simulink model "EV_powertrain"  (R2018a)
settings: Solver=FixedStepAuto  StartTime=0.0  StopTime=10.5  FixedStep=0.1  MaxStep=19.86  RelTol=1e-3
values from neighbouring files (symbols this model uses):
  A = 3.8065    [artemisUrban_drive_cycle.m]
  cd = 0.28    [artemisUrban_drive_cycle.m]
  crf = 0.015    [artemisUrban_drive_cycle.m]
  GR = 7.9377    [artemisUrban_drive_cycle.m]
  GVM = M+Md    (= 1710.665)    [artemisUrban_drive_cycle.m]
  GVW = GVM*g    (= 16781.62365)    [artemisUrban_drive_cycle.m]
  MCE_Eff = MCE(:,2:16)    [artemisUrban_drive_cycle.m]
  MCE_Speed = MCE(:,1)    [artemisUrban_drive_cycle.m]
  MCE_Torque = MCE(:,17)    [artemisUrban_drive_cycle.m]
  MCRE_Eff = MCRE(:,2:16)    [artemisUrban_drive_cycle.m]
  MCRE_Speed = MCRE(:,1)    [artemisUrban_drive_cycle.m]
  MCRE_Torque = MCRE(:,17)    [artemisUrban_drive_cycle.m]
  ME_Eff = ME(:,2:16)    [artemisUrban_drive_cycle.m]
  ME_Speed = ME(:,1)    [artemisUrban_drive_cycle.m]
  ME_Torque = ME(:,17)    [artemisUrban_drive_cycle.m]
  MRE_Eff = MRE(:,2:16)    [artemisUrban_drive_cycle.m]
  MRE_Speed = MRE(:,1)    [artemisUrban_drive_cycle.m]
  MRE_Torque = MRE(:,17)    [artemisUrban_drive_cycle.m]
  rho = 1.2250    (= 1.225)    [artemisUrban_drive_cycle.m]
  Rw = 0.2032    [artemisUrban_drive_cycle.m]
  Teff = 0.89    [artemisUrban_drive_cycle.m]
settings Model: Creator=VAISHNAV  LastModifiedBy=VAISHNAV

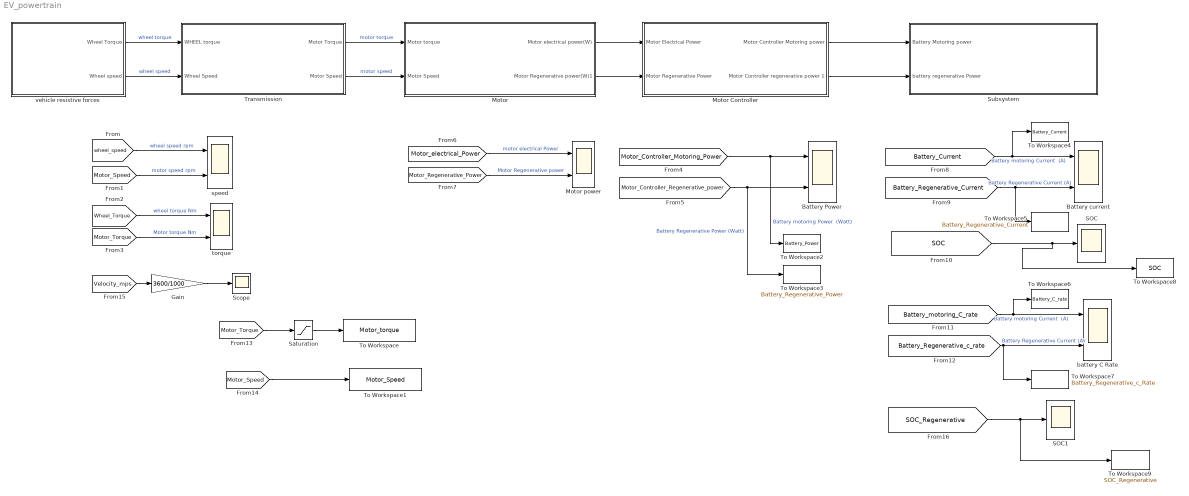
== system EV_powertrain ==
  Battery Power : Scope  NumInputPorts=2
  "Battery current " : Scope  NumInputPorts=2
  Gain : Gain  Gain=3600/1000
  "Motor " : Subsystem
  Motor Controller : Subsystem
  Motor power : Scope  NumInputPorts=2
  SOC : Scope
  SOC1 : Scope
  Saturation : Saturate  UpperLimit=inf  LowerLimit=0
  Scope : Scope
  Subsystem : Subsystem
  To Workspace : ToWorkspace  VariableName=Motor_torque  SaveFormat=Timeseries  SampleTime=-1
  To Workspace1 : ToWorkspace  VariableName=Motor_Speed  SaveFormat=Timeseries  SampleTime=-1
  To Workspace2 : ToWorkspace  VariableName=Battery_Power  SaveFormat=Timeseries  SampleTime=-1
  To Workspace3 : ToWorkspace  VariableName=Battery_Regenerative_Power  SaveFormat=Timeseries  SampleTime=-1
  To Workspace4 : ToWorkspace  VariableName=Battery_Current  SaveFormat=Timeseries  SampleTime=-1
  To Workspace5 : ToWorkspace  VariableName=Battery_Regenerative_Current  SaveFormat=Timeseries  SampleTime=-1
  To Workspace6 : ToWorkspace  VariableName=Battery_C_rate  SaveFormat=Timeseries  SampleTime=-1
  To Workspace7 : ToWorkspace  VariableName=Battery_Regenerative_c_Rate  SaveFormat=Timeseries  SampleTime=-1
  To Workspace8 : ToWorkspace  VariableName=SOC  SaveFormat=Timeseries  SampleTime=-1
  To Workspace9 : ToWorkspace  VariableName=SOC_Regenerative  SaveFormat=Timeseries  SampleTime=-1
  Transmission : Subsystem
  battery C Rate : Scope  NumInputPorts=2
  speed : Scope  NumInputPorts=2
  torque : Scope  NumInputPorts=2
  vehicle resistive forces : Subsystem
  wires:
  vehicle resistive forces/1(Wheel Torque) -> Transmission/1(WHEEL torque)  "wheel torque"
  vehicle resistive forces/2(Wheel speed) -> Transmission/2(Wheel Speed)  "wheel speed"
  [wheel_speed] -> speed/1  "wheel speed rpm"
  [Motor_Speed] -> speed/2  "motor speed rpm"
  [Wheel_Torque] -> torque/1  "wheel torque Nm"
  [Motor_Torque] -> torque/2  "Motor torque Nm"
  Transmission/1(Motor Torque) -> "Motor "/1(Motor torque)  "motor torque"
  Transmission/2(Motor Speed) -> "Motor "/2(Motor Speed)  "motor speed"
  [Motor_electrical_Power] -> Motor power/1  "motor electrical Power"
  [Motor_Regenerative_Power] -> Motor power/2  "Motor Regenerative power"
  "Motor "/1(Motor electrical power(W)) -> Motor Controller/1(Motor Electrical Power)
  "Motor "/2(Motor Regenerative power(W)1) -> Motor Controller/2(Motor Regenerative Power)
  [Motor_Controller_Motoring_Power] -> To Workspace2/1, Battery Power/1  "Battery motoring Power  (Watt)"
  [Motor_Controller_Regenerative_power] -> To Workspace3/1, Battery Power/2  "Battery Regenerative Power (Watt)"
  [Battery_Current] -> To Workspace4/1, "Battery current "/1  "Battery motoring Current  (A)"
  [Battery_Regenerative_Current] -> To Workspace5/1, "Battery current "/2  "Battery Regenerative Current (A)"
  [SOC] -> To Workspace8/1, SOC/1
  [Battery_Regenerative_c_rate] -> To Workspace7/1, battery C Rate/2  "Battery Regenerative Current (A)"
  [Battery_motoring_C_rate] -> To Workspace6/1, battery C Rate/1  "Battery motoring Current  (A)"
  Saturation/1 -> To Workspace/1
  [Motor_Torque] -> Saturation/1
  [Motor_Speed] -> To Workspace1/1
  [Velocity_mps] -> Gain/1
  Gain/1 -> Scope/1
  [SOC_Regenerative] -> To Workspace9/1, SOC1/1
  Motor Controller/2(Motor Controller regenerative power 1) -> Subsystem/2(battery regenerative Power)
  Motor Controller/1("Motor Controller Motoring power ") -> Subsystem/1(Battery Motoring power)

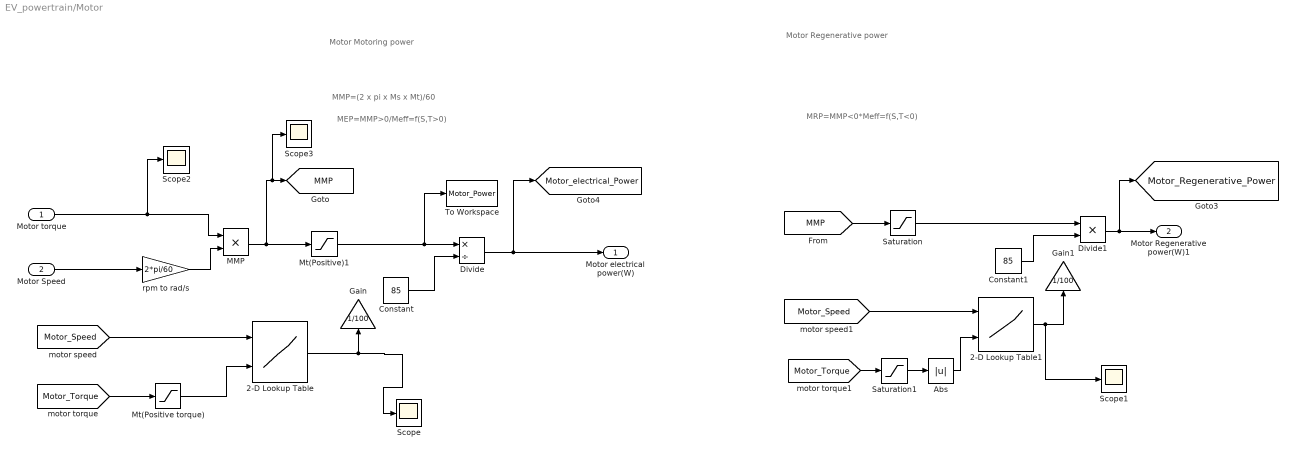
== system EV_powertrain/Motor  ==
  note: MRP=MMP<0*Meff=f(S,T<0)
  note: Motor Regenerative power
  note: MEP=MMP>0/Meff=f(S,T>0)
  note: MMP=(2 x pi x Ms x Mt)/60
  note: Motor Motoring power
  Motor torque : Inport
  Motor Speed : Inport  Port=2
  2-D Lookup Table : Lookup_n-D  BreakpointsForDimension1=ME_Speed  BreakpointsForDimension2=ME_Torque  Table=ME_Eff  InternalRulePriority=Speed  RndMeth=Simplest  InputSameDT=on
  2-D Lookup Table1 : Lookup_n-D  BreakpointsForDimension1=MRE_Speed  BreakpointsForDimension2=MRE_Torque  Table=MRE_Eff  InternalRulePriority=Speed  RndMeth=Simplest  InputSameDT=on
  Abs : Abs
  Constant : Constant  Value=85
  Constant1 : Constant  Value=85
  Divide : Product  Inputs=*/
  Divide1 : Product  Inputs=**
  Gain : Gain  Gain=1/100
  Gain1 : Gain  Gain=1/100
  MMP : Product
  Mt(Positive torque) : Saturate  UpperLimit=inf  LowerLimit=0
  Mt(Positive)1 : Saturate  UpperLimit=inf  LowerLimit=0
  Saturation : Saturate  UpperLimit=0  LowerLimit=-inf
  Saturation1 : Saturate  UpperLimit=0  LowerLimit=-inf
  Scope{,1..3} (4 alike) : Scope
  To Workspace : ToWorkspace  VariableName=Motor_Power  SaveFormat=Timeseries  SampleTime=-1
  rpm to rad/s : Gain  Gain=2*pi/60
  Motor electrical power(W) : Outport
  Motor Regenerative power(W)1 : Outport  Port=2
  tag scope: MMP=global, Motor_Regenerative_Power=global, Motor_electrical_Power=global
  wires:
  Motor Speed/1 -> rpm to rad/s/1
  Motor torque/1 -> Scope2/1, MMP/1
  rpm to rad/s/1 -> MMP/2
  [Motor_Speed] -> 2-D Lookup Table/1
  Mt(Positive torque)/1 -> 2-D Lookup Table/2
  [Motor_Torque] -> Mt(Positive torque)/1
  MMP/1 -> Scope3/1, [MMP], Mt(Positive)1/1
  Divide/1 -> [Motor_electrical_Power], Motor electrical power(W)/1
  Mt(Positive)1/1 -> To Workspace/1, Divide/1
  [MMP] -> Saturation/1
  [Motor_Torque] -> Saturation1/1
  [Motor_Speed] -> 2-D Lookup Table1/1
  2-D Lookup Table1/1 -> Scope1/1, Gain1/1
  Saturation/1 -> Divide1/1
  Saturation1/1 -> Abs/1
  Abs/1 -> 2-D Lookup Table1/2
  Divide1/1 -> [Motor_Regenerative_Power], Motor Regenerative power(W)1/1
  2-D Lookup Table/1 -> Scope/1, Gain/1
  Constant/1 -> Divide/2
  Constant1/1 -> Divide1/2

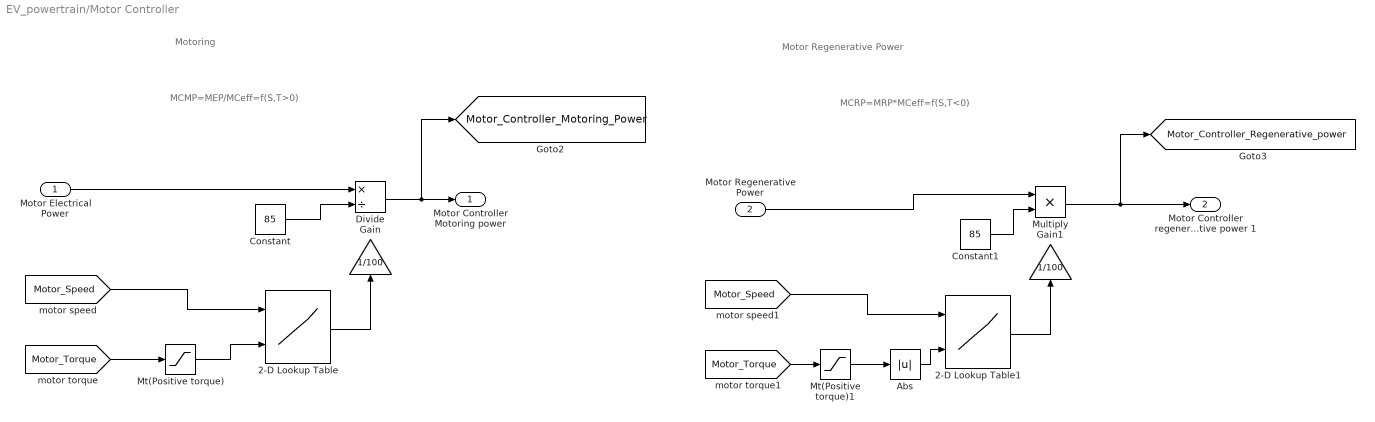
== system EV_powertrain/Motor Controller ==
  note: MCRP=MRP*MCeff=f(S,T<0)
  note: Motor Regenerative Power
  note: MCMP=MEP/MCeff=f(S,T>0)
  note: Motoring
  Motor Electrical Power : Inport
  Motor Regenerative Power : Inport  Port=2
  2-D Lookup Table : Lookup_n-D  BreakpointsForDimension1=MCE_Speed  BreakpointsForDimension2=MCE_Torque  Table=MCE_Eff  InternalRulePriority=Speed  RndMeth=Simplest  InputSameDT=on
  2-D Lookup Table1 : Lookup_n-D  BreakpointsForDimension1=MCRE_Speed  BreakpointsForDimension2=MCRE_Torque  Table=MCRE_Eff  InternalRulePriority=Speed  RndMeth=Simplest  InputSameDT=on
  Abs : Abs
  Constant : Constant  Value=85
  Constant1 : Constant  Value=85
  Divide : Product  Inputs=*/
  Gain : Gain  Gain=1/100
  Gain1 : Gain  Gain=1/100
  Mt(Positive torque) : Saturate  UpperLimit=inf  LowerLimit=0
  Mt(Positive torque)1 : Saturate  UpperLimit=0  LowerLimit=-inf
  Multiply : Product
  "Motor Controller Motoring power " : Outport
  Motor Controller regenerative power 1 : Outport  Port=2
  tag scope: Motor_Controller_Motoring_Power=global, Motor_Controller_Regenerative_power=global
  wires:
  [Motor_Torque] -> Mt(Positive torque)/1
  [Motor_Speed] -> 2-D Lookup Table/1
  Mt(Positive torque)/1 -> 2-D Lookup Table/2
  2-D Lookup Table/1 -> Gain/1
  Motor Electrical Power/1 -> Divide/1
  Divide/1 -> [Motor_Controller_Motoring_Power], "Motor Controller Motoring power "/1
  [Motor_Speed] -> 2-D Lookup Table1/1
  [Motor_Torque] -> Mt(Positive torque)1/1
  2-D Lookup Table1/1 -> Gain1/1
  Motor Regenerative Power/1 -> Multiply/1
  Multiply/1 -> [Motor_Controller_Regenerative_power], Motor Controller regenerative power 1/1
  Mt(Positive torque)1/1 -> Abs/1
  Abs/1 -> 2-D Lookup Table1/2
  Constant/1 -> Divide/2
  Constant1/1 -> Multiply/2

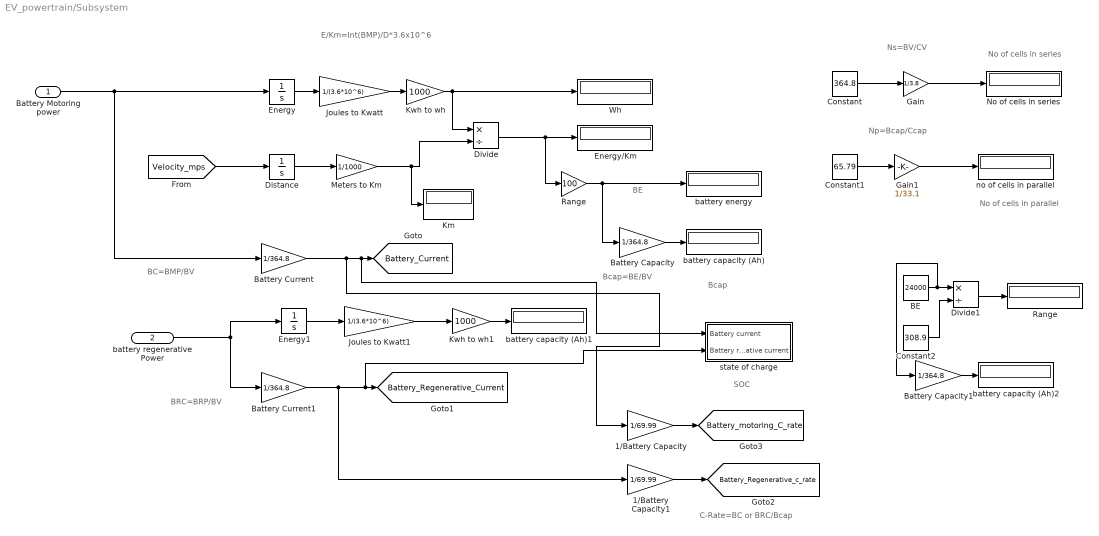
== system EV_powertrain/Subsystem ==
  note: BC=BMP/BV
  note: Bcap
  note: BE
  note: No of cells in parallel
  note: No of cells in series
  note: C-Rate=BC or BRC/Bcap
  note: SOC
  note: Np=Bcap/Ccap
  note: Ns=BV/CV
  note: Bcap=BE/BV
  note: E/Km=Int(BMP)/D*3.6x10^6
  note: BRC=BRP/BV
  Battery Motoring power : Inport
  battery regenerative Power : Inport  Port=2
  1/Battery Capacity : Gain  Gain=1/69.99
  1/Battery Capacity1 : Gain  Gain=1/69.99
  BE : Constant  Value=24000
  Battery Capacity : Gain  Gain=1/364.8
  Battery Capacity1 : Gain  Gain=1/364.8
  Battery Current : Gain  Gain=1/364.8
  Battery Current1 : Gain  Gain=1/364.8
  Constant : Constant  Value=364.8
  Constant1 : Constant  Value=65.79
  Constant2 : Constant  Value=308.9
  Distance : Integrator
  Divide : Product  Inputs=*/
  Divide1 : Product  Inputs=*/
  Energy : Integrator
  Energy/Km : Display
  Energy1 : Integrator
  Gain : Gain  Gain=1/3.8
  Gain1 : Gain  Gain=1/33.1
  Joules to Kwatt : Gain  Gain=1/(3.6*10^6)
  Joules to Kwatt1 : Gain  Gain=1/(3.6*10^6)
  Km : Display
  Kwh to wh : Gain  Gain=1000
  Kwh to wh1 : Gain  Gain=1000
  Meters to Km : Gain  Gain=1/1000
  No of cells in series : Display
  Range : Gain  Gain=100
  "Range " : Display
  Wh : Display
  battery capacity (Ah) : Display
  battery capacity (Ah)1 : Display
  battery capacity (Ah)2 : Display
  battery energy : Display
  no of cells in parallel : Display
  state of charge : Subsystem
  tag scope: Battery_Current=global, Battery_Regenerative_Current=global, Battery_Regenerative_c_rate=global, Battery_motoring_C_rate=global
  wires:
  Battery Motoring power/1 -> Energy/1, Battery Current/1
  [Velocity_mps] -> Distance/1
  Energy/1 -> Joules to Kwatt/1
  Joules to Kwatt/1 -> Kwh to wh/1
  Kwh to wh/1 -> Wh/1, Divide/1
  Divide/1 -> Range/1, Energy/Km/1
  Distance/1 -> Meters to Km/1
  Meters to Km/1 -> Km/1, Divide/2
  Range/1 -> Battery Capacity/1, battery energy/1
  Battery Capacity/1 -> battery capacity (Ah)/1
  battery regenerative Power/1 -> Energy1/1, Battery Current1/1
  Battery Current1/1 -> 1/Battery Capacity1/1, state of charge/2("Battery regenerative current "), [Battery_Regenerative_Current]
  Energy1/1 -> Joules to Kwatt1/1
  Joules to Kwatt1/1 -> Kwh to wh1/1
  Kwh to wh1/1 -> battery capacity (Ah)1/1
  Gain/1 -> No of cells in series/1
  Constant/1 -> Gain/1
  Constant1/1 -> Gain1/1
  Gain1/1 -> no of cells in parallel/1
  1/Battery Capacity/1 -> [Battery_motoring_C_rate]
  1/Battery Capacity1/1 -> [Battery_Regenerative_c_rate]
  Constant2/1 -> Divide1/2
  BE/1 -> Battery Capacity1/1, Divide1/1
  Divide1/1 -> "Range "/1
  Battery Capacity1/1 -> battery capacity (Ah)2/1
  Battery Current/1 -> 1/Battery Capacity/1, state of charge/1(Battery current), [Battery_Current]

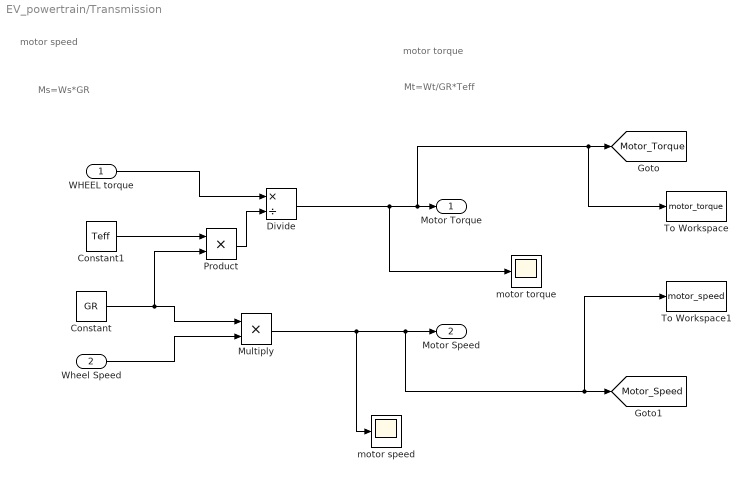
== system EV_powertrain/Transmission ==
  note: Mt=Wt/GR*Teff
  note: Ms=Ws*GR
  note: motor torque
  note: motor speed
  WHEEL torque : Inport
  Wheel Speed : Inport  Port=2
  Constant : Constant  Value=GR
  Constant1 : Constant  Value=Teff
  Divide : Product  Inputs=*/
  Multiply : Product
  Product : Product
  To Workspace : ToWorkspace  VariableName=motor_torque  SaveFormat=Timeseries  SampleTime=-1
  To Workspace1 : ToWorkspace  VariableName=motor_speed  SaveFormat=Timeseries  SampleTime=-1
  motor speed : Scope
  motor torque : Scope
  Motor Torque : Outport
  Motor Speed : Outport  Port=2
  tag scope: Motor_Speed=global, Motor_Torque=global
  wires:
  Wheel Speed/1 -> Multiply/2
  Constant/1 -> Product/2, Multiply/1
  Multiply/1 -> motor speed/1, To Workspace1/1, [Motor_Speed], Motor Speed/1
  Divide/1 -> motor torque/1, To Workspace/1, [Motor_Torque], Motor Torque/1
  Constant1/1 -> Product/1
  Product/1 -> Divide/2
  WHEEL torque/1 -> Divide/1

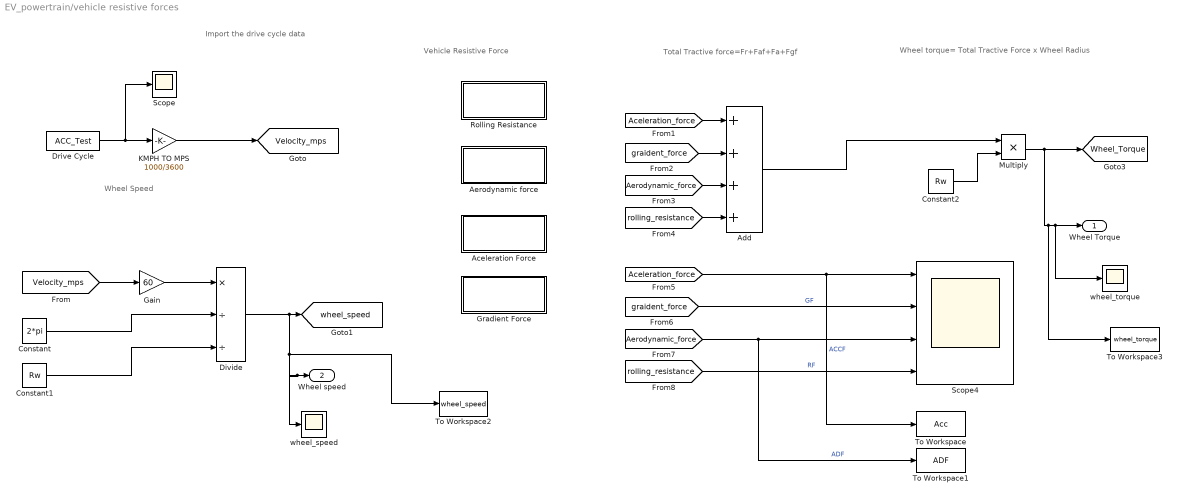
== system EV_powertrain/vehicle resistive forces ==
  note: Wheel torque= Total Tractive Force x Wheel Radius
  note: Total Tractive force=Fr+Faf+Fa+Fgf
  note: Vehicle Resistive Force
  note: Wheel Speed
  note: Import the drive cycle data
  Aceleration Force : Subsystem
  Add : Sum  Inputs=++++
  Aerodynamic force : Subsystem
  Constant : Constant  Value=2*pi
  Constant1 : Constant  Value=Rw
  Constant2 : Constant  Value=Rw
  Divide : Product  Inputs=*//
  Drive Cycle : FromWorkspace  VariableName=ACC_Test  SampleTime=0
  Gain : Gain  Gain=60
  Gradient Force : Subsystem
  KMPH TO MPS : Gain  Gain=1000/3600
  Multiply : Product
  Rolling Resistance : Subsystem
  Scope : Scope
  Scope4 : Scope  NumInputPorts=4
  To Workspace : ToWorkspace  VariableName=Acc  SaveFormat=Timeseries  SampleTime=-1
  To Workspace1 : ToWorkspace  VariableName=ADF  SaveFormat=Timeseries  SampleTime=-1
  To Workspace2 : ToWorkspace  VariableName=wheel_speed  SaveFormat=Timeseries  SampleTime=-1
  To Workspace3 : ToWorkspace  VariableName=wheel_torque  SaveFormat=Timeseries  SampleTime=-1
  wheel_speed : Scope
  wheel_torque : Scope
  Wheel Torque : Outport
  Wheel speed : Outport  Port=2
  tag scope: Velocity_mps=global, Wheel_Torque=global, wheel_speed=global
  wires:
  Drive Cycle/1 -> Scope/1, KMPH TO MPS/1
  KMPH TO MPS/1 -> [Velocity_mps]
  [Velocity_mps] -> Gain/1
  Gain/1 -> Divide/1
  Constant/1 -> Divide/2
  Constant1/1 -> Divide/3
  Divide/1 -> To Workspace2/1, wheel_speed/1, Wheel speed/1, [wheel_speed]
  Constant2/1 -> Multiply/2
  Multiply/1 -> To Workspace3/1, wheel_torque/1, Wheel Torque/1, [Wheel_Torque]
  [Aceleration_force] -> Add/1
  [graident_force] -> Add/2
  [Aerodynamic_force] -> Add/3
  [rolling_resistance] -> Add/4
  Add/1 -> Multiply/1
  [Aceleration_force] -> To Workspace/1, Scope4/1  "ACCF"
  [graident_force] -> Scope4/2  "GF"
  [Aerodynamic_force] -> To Workspace1/1, Scope4/3  "ADF"
  [rolling_resistance] -> Scope4/4  "RF"

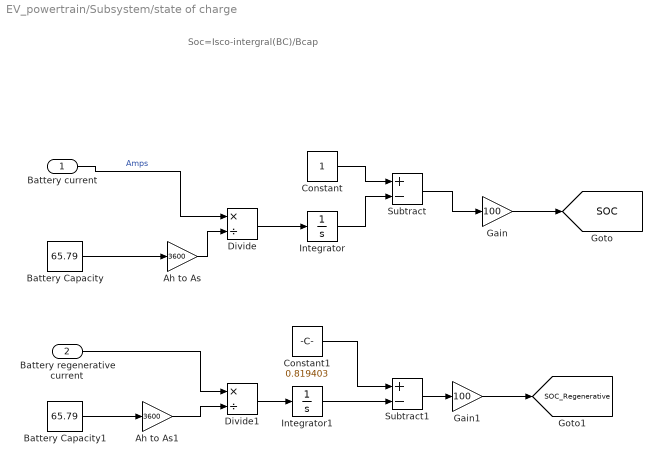
== system EV_powertrain/Subsystem/state of charge ==
  note: Soc=Isco-intergral(BC)/Bcap
  Battery current : Inport
  "Battery regenerative current " : Inport  Port=2
  Ah to As : Gain  Gain=3600
  Ah to As1 : Gain  Gain=3600
  Battery Capacity : Constant  Value=65.79
  Battery Capacity1 : Constant  Value=65.79
  Constant : Constant
  Constant1 : Constant  Value=0.819403
  Divide : Product  Inputs=*/
  Divide1 : Product  Inputs=*/
  Gain : Gain  Gain=100
  Gain1 : Gain  Gain=100
  Integrator : Integrator
  Integrator1 : Integrator
  Subtract : Sum  Inputs=+-
  Subtract1 : Sum  Inputs=+-
  tag scope: SOC=global, SOC_Regenerative=global
  wires:
  Ah to As/1 -> Divide/2
  Battery Capacity/1 -> Ah to As/1
  Battery current/1 -> Divide/1  "Amps"
  Divide/1 -> Integrator/1
  Gain/1 -> [SOC]
  Integrator/1 -> Subtract/2
  Constant/1 -> Subtract/1
  Subtract/1 -> Gain/1
  Battery Capacity1/1 -> Ah to As1/1
  Ah to As1/1 -> Divide1/2
  "Battery regenerative current "/1 -> Divide1/1
  Divide1/1 -> Integrator1/1
  Integrator1/1 -> Subtract1/2
  Constant1/1 -> Subtract1/1
  Subtract1/1 -> Gain1/1
  Gain1/1 -> [SOC_Regenerative]

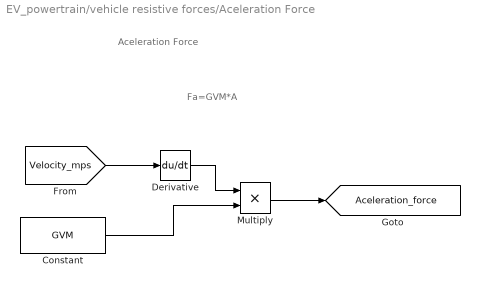
== system EV_powertrain/vehicle resistive forces/Aceleration Force ==
  note: Fa=GVM*A
  note: Aceleration Force
  Constant : Constant  Value=GVM
  Derivative : Derivative
  Multiply : Product
  tag scope: Aceleration_force=global
  wires:
  Constant/1 -> Multiply/2
  Multiply/1 -> [Aceleration_force]
  [Velocity_mps] -> Derivative/1
  Derivative/1 -> Multiply/1

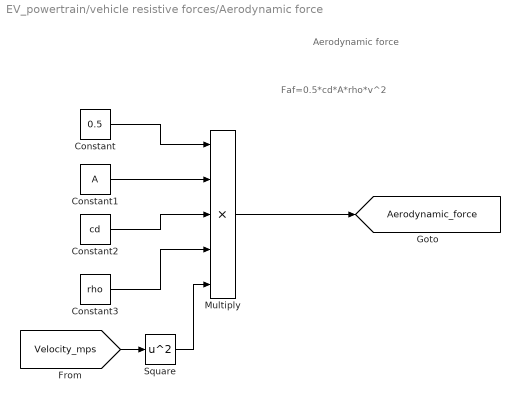
== system EV_powertrain/vehicle resistive forces/Aerodynamic force ==
  note: Faf=0.5*cd*A*rho*v^2
  note: Aerodynamic force
  Constant : Constant  Value=0.5
  Constant1 : Constant  Value=A
  Constant2 : Constant  Value=cd
  Constant3 : Constant  Value=rho
  Multiply : Product  Inputs=5
  Square : Math  Operator=square  SaturateOnIntegerOverflow=on
  tag scope: Aerodynamic_force=global
  wires:
  Constant/1 -> Multiply/1
  Constant1/1 -> Multiply/2
  Constant2/1 -> Multiply/3
  Constant3/1 -> Multiply/4
  Multiply/1 -> [Aerodynamic_force]
  [Velocity_mps] -> Square/1
  Square/1 -> Multiply/5

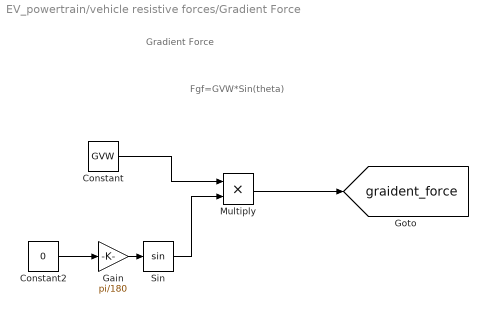
== system EV_powertrain/vehicle resistive forces/Gradient Force ==
  note: Fgf=GVW*Sin(theta)
  note: Gradient Force
  Constant : Constant  Value=GVW
  Constant2 : Constant  Value=0
  Gain : Gain  Gain=pi/180
  Multiply : Product
  Sin : Trigonometry
  tag scope: graident_force=global
  wires:
  Multiply/1 -> [graident_force]
  Constant/1 -> Multiply/1
  Sin/1 -> Multiply/2
  Gain/1 -> Sin/1
  Constant2/1 -> Gain/1

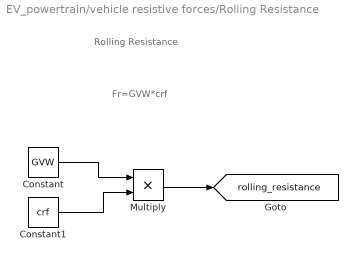
== system EV_powertrain/vehicle resistive forces/Rolling Resistance ==
  note: Fr=GVW*crf
  note: Rolling Resistance
  Constant : Constant  Value=GVW
  Constant1 : Constant  Value=crf
  Multiply : Product
  tag scope: rolling_resistance=global
  wires:
  Constant/1 -> Multiply/1
  Constant1/1 -> Multiply/2
  Multiply/1 -> [rolling_resistance]
